simulink model "ProyectooModelado"  (R2024b)
settings: Solver=ode23s  StartTime=0.0  StopTime=30.0  MaxStep=1e-3  RelTol=1e-3
libraries: slpidlib x1
settings Model: Creator=Nicole Elias
settings DataIOCC: ReturnWorkspaceOutputs=off  TimeSaveName=t
settings DebuggingCC: AlgebraicLoopMsg=none  ArtificialAlgebraicLoopMsg=none  InheritedTsInSrcMsg=none  OperatingPointInterfaceChecksumMismatchMsg=none
settings RTWCC: GPUComputeCapability=3.5

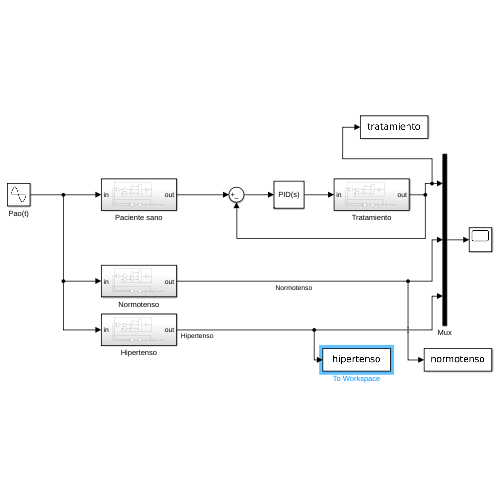
[thumbnail: Simulink's stored preview of the top-level diagram]
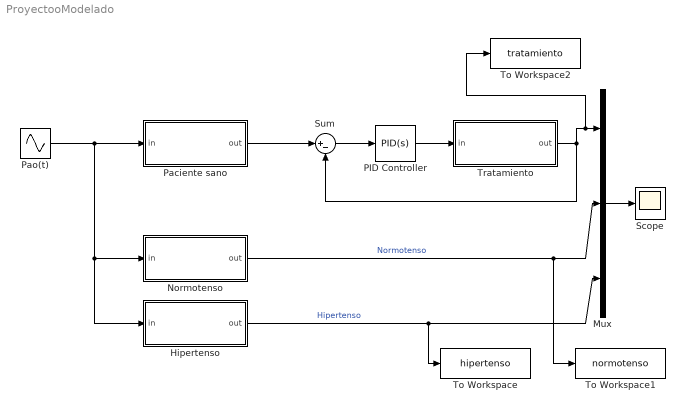
== system ProyectooModelado ==
  Hipertenso : Subsystem
  Mux : Mux  Inputs=3
  Normotenso : Subsystem
  PID Controller : slpidlib/PID Controller  Controller=PID  Form=Parallel  TimeDomain=Continuous-time  UseExternalTs=off  SampleTime=-1  IntegratorMethod=Forward Euler  FilterMethod=Forward Euler  ControllerParametersSource=internal  P=339.126  I=9679.425  UseKiTs=off  D=0.3924  UseExternalDerivativeSource=off  N=100  UseFilter=on  TunerSelectOption=Transfer Function Based (PID Tuner App)  InitialConditionSource=internal  InitialConditionForIntegrator=0  InitialConditionForFilter=0  DifferentiatorICPrevScaledInput=0  ExternalReset=none  TrackingMode=off  Kt=1  LimitOutput=off  SatLimitsSource=internal  UpperSaturationLimit=inf  LowerSaturationLimit=-inf  LinearizeAsGain=on  AntiWindupMode=none  Kb=1  LimitIntegrator=off  UpperIntegratorSaturationLimit=inf  LowerIntegratorSaturationLimit=-inf  POutMin=[]  POutMax=[]  IOutMin=[]  IOutMax=[]  DOutMin=[]  DOutMax=[]  NOutMin=[]  NOutMax=[]  SumOutMin=[]  SumOutMax=[]  SaturationOutMin=[]  SaturationOutMax=[]  PParamMin=[]  PParamMax=[]  IParamMin=[]  IParamMax=[]  DParamMin=[]  DParamMax=[]  NParamMin=[]  NParamMax=[]  KbParamMin=[]  KbParamMax=[]  KtParamMin=[]  KtParamMax=[]  KbOutMin=[]  KbOutMax=[]  KtOutMin=[]  KtOutMax=[]  IntegratorOutMin=[]  IntegratorOutMax=[]  FilterOutMin=[]  FilterOutMax=[]  SumI1OutMin=[]  SumI1OutMax=[]  SumI2OutMin=[]  SumI2OutMax=[]  SumI3OutMin=[]  SumI3OutMax=[]  SumI4OutMin=[]  SumI4OutMax=[]  SumDOutMin=[]  SumDOutMax=[]  DifferentiatorOutMin=[]  DifferentiatorOutMax=[]  FilterDiffOutCoefMin=[]  FilterDiffOutCoefMax=[]  ReciprocalOutMin=[]  ReciprocalOutMax=[]  SumDenOutMin=[]  SumDenOutMax=[]  SumNumOutMin=[]  SumNumOutMax=[]  DivideOutMin=[]  DivideOutMax=[]  UdiffTsProdOutMin=[]  UdiffTsProdOutMax=[]  NTsProdOutMin=[]  NTsProdOutMax=[]  UintegralTsProdOutMin=[]  UintegralTsProdOutMax=[]  UngainTsProdOutMin=[]  UngainTsProdOutMax=[]  ClampingZeroOutDataTypeStr=Inherit: Inherit via back propagation  ClampingZeroOutMin=[]  ClampingZeroOutMax=[]  FilterDenConstantOutDataTypeStr=Inherit: Inherit via back propagation  FilterDenConstantOutMin=[]  FilterDenConstantOutMax=[]  PCopyOutDataTypeStr=Inherit: Inherit via back propagation  PCopyOutMin=[]  PCopyOutMax=[]  NCopyOutDataTypeStr=Inherit: Inherit via back propagation  NCopyOutMin=[]  NCopyOutMax=[]  IntegratorContinuousStateAttributes=''  IntegratorStateMustResolveToSignalObject=off  IntegratorRTWStateStorageClass=Auto  FilterContinuousStateAttributes=''  FilterStateMustResolveToSignalObject=off  FilterRTWStateStorageClass=Auto  ParallelPVariant=InternalParameters  IdealPVariant=Disabled  IVariant=InternalParameters  DVariant=InternalParameters  IntegratorVariant=Continuous  SatVariant=Disabled  AWVariant=Passthrough  PCopyVariant=Disabled  TRVariant=Disabled  FdbkBlocksVariant=Forward  IdealPFdbkVariant=Disabled  SatFdbkVariant=Disabled  DerivativeFilterVariant=ContFilter  NVariant=InternalParameters  NCopyVariant=Disabled  FilterICVariant=InternalICsFilter  IntegratorICVariant=InternalICs  ExternalResetVariant=Disabled  TRSumVariant=Passthrough  SumFdbkVariant=Disabled  SumVariant=Sum_PID  TsampFilterVariant=InternalTs  TsampNgainVariant=Passthrough  TsampIntegralVariant=Disabled_SignalSpec  ExternalSaturationOutDataTypeStr=Inherit: Same as second input  DerivativeSourceVariant=ErrorSignal  PreIntVariant=InternalPreInt
  Paciente sano : Subsystem
  Pao(t) : Sin  Amplitude=2.5  Frequency=1.5707
  Scope : Scope
  Sum : Sum  Inputs=|+-
  To Workspace : ToWorkspace  VariableName=hipertenso  SaveFormat=Structure With Time  SampleTime=-1
  To Workspace1 : ToWorkspace  VariableName=normotenso  SaveFormat=Structure With Time  SampleTime=-1
  To Workspace2 : ToWorkspace  VariableName=tratamiento  SaveFormat=Structure With Time  SampleTime=-1
  Tratamiento : Subsystem
  wires:
  Pao(t)/1 -> Paciente sano/1(in), Hipertenso/1(in), Normotenso/1(in)
  Paciente sano/1(out) -> Sum/1
  Normotenso/1(out) -> To Workspace1/1, Mux/2  "Normotenso"
  Mux/1 -> Scope/1
  Sum/1 -> PID Controller/1
  Tratamiento/1(out) -> Sum/2, To Workspace2/1, Mux/1
  PID Controller/1 -> Tratamiento/1(in)
  Hipertenso/1(out) -> To Workspace/1, Mux/3  "Hipertenso"

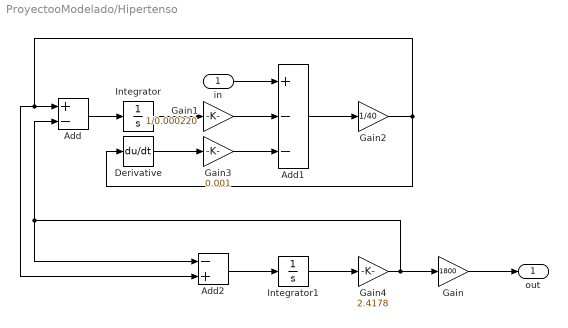
== system ProyectooModelado/Hipertenso ==
  in : Inport
  Add : Sum  Inputs=+-
  Add1 : Sum  Inputs=+--
  Add2 : Sum  Inputs=-+
  Derivative : Derivative
  Gain : Gain  Gain=1800
  Gain1 : Gain  Gain=1/0.000220
  Gain2 : Gain  Gain=1/40
  Gain3 : Gain  Gain=0.001
  Gain4 : Gain  Gain=2.4178
  Integrator : Integrator
  Integrator1 : Integrator
  out : Outport
  wires:
  Add/1 -> Integrator/1
  Integrator/1 -> Gain1/1
  Gain1/1 -> Add1/2
  Add1/1 -> Gain2/1
  in/1 -> Add1/1
  Gain2/1 -> Derivative/1, Add/1, Add2/2
  Derivative/1 -> Gain3/1
  Gain3/1 -> Add1/3
  Integrator1/1 -> Gain4/1
  Add2/1 -> Integrator1/1
  Gain4/1 -> Gain/1, Add/2, Add2/1
  Gain/1 -> out/1

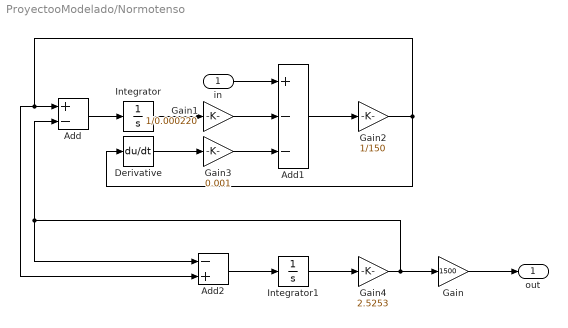
== system ProyectooModelado/Normotenso ==
  in : Inport
  Add : Sum  Inputs=+-
  Add1 : Sum  Inputs=+--
  Add2 : Sum  Inputs=-+
  Derivative : Derivative
  Gain : Gain  Gain=1500
  Gain1 : Gain  Gain=1/0.000220
  Gain2 : Gain  Gain=1/150
  Gain3 : Gain  Gain=0.001
  Gain4 : Gain  Gain=2.5253
  Integrator : Integrator
  Integrator1 : Integrator
  out : Outport
  wires:
  Add/1 -> Integrator/1
  Integrator/1 -> Gain1/1
  Gain1/1 -> Add1/2
  Add1/1 -> Gain2/1
  in/1 -> Add1/1
  Gain2/1 -> Derivative/1, Add/1, Add2/2
  Derivative/1 -> Gain3/1
  Gain3/1 -> Add1/3
  Integrator1/1 -> Gain4/1
  Add2/1 -> Integrator1/1
  Gain4/1 -> Gain/1, Add/2, Add2/1
  Gain/1 -> out/1

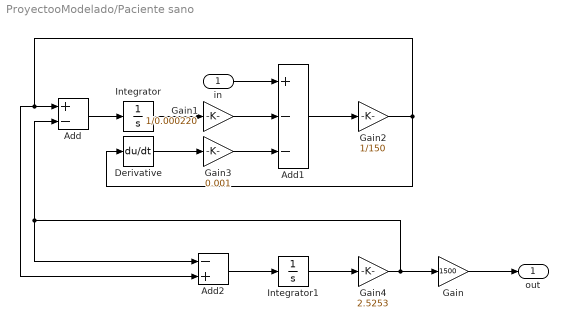
== system ProyectooModelado/Paciente sano ==
  in : Inport
  Add : Sum  Inputs=+-
  Add1 : Sum  Inputs=+--
  Add2 : Sum  Inputs=-+
  Derivative : Derivative
  Gain : Gain  Gain=1500
  Gain1 : Gain  Gain=1/0.000220
  Gain2 : Gain  Gain=1/150
  Gain3 : Gain  Gain=0.001
  Gain4 : Gain  Gain=2.5253
  Integrator : Integrator
  Integrator1 : Integrator
  out : Outport
  wires:
  Add/1 -> Integrator/1
  Integrator/1 -> Gain1/1
  Gain1/1 -> Add1/2
  Add1/1 -> Gain2/1
  in/1 -> Add1/1
  Gain2/1 -> Derivative/1, Add/1, Add2/2
  Derivative/1 -> Gain3/1
  Gain3/1 -> Add1/3
  Integrator1/1 -> Gain4/1
  Add2/1 -> Integrator1/1
  Gain4/1 -> Gain/1, Add/2, Add2/1
  Gain/1 -> out/1

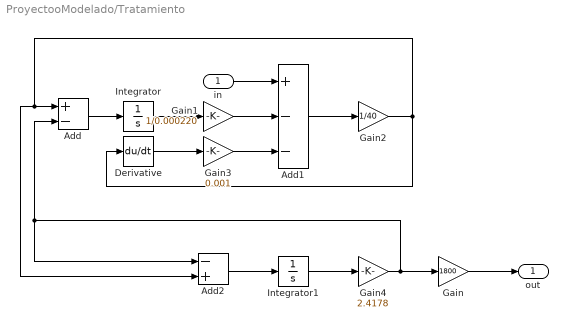
== system ProyectooModelado/Tratamiento ==
  in : Inport
  Add : Sum  Inputs=+-
  Add1 : Sum  Inputs=+--
  Add2 : Sum  Inputs=-+
  Derivative : Derivative
  Gain : Gain  Gain=1800
  Gain1 : Gain  Gain=1/0.000220
  Gain2 : Gain  Gain=1/40
  Gain3 : Gain  Gain=0.001
  Gain4 : Gain  Gain=2.4178
  Integrator : Integrator
  Integrator1 : Integrator
  out : Outport
  wires:
  Add/1 -> Integrator/1
  Integrator/1 -> Gain1/1
  Gain1/1 -> Add1/2
  Add1/1 -> Gain2/1
  in/1 -> Add1/1
  Gain2/1 -> Derivative/1, Add/1, Add2/2
  Derivative/1 -> Gain3/1
  Gain3/1 -> Add1/3
  Integrator1/1 -> Gain4/1
  Add2/1 -> Integrator1/1
  Gain4/1 -> Gain/1, Add/2, Add2/1
  Gain/1 -> out/1
